simulink model "vehicle_steering"  (R2022a)
settings: Solver=VariableStepAuto  StartTime=0.0  StopTime=10  RelTol=1e-3
model workspace (MATLAB code in the model file):
  | a = 0.5;
  | b = 1;
  | A = [0, 1; 0, 0];
  | B = [a/b; 1];
  | C = [1, 0];
  | D = 0;
  | 
  | P = [-5, -5];
  | % P = [-50, -50];
  | 
  | kr = 23;
  | % kr = 2300;
  | % kr = 90;
  | K = acker(A, B, P);
  | L = [100; 1000]; % from hit and trial
settings Model: Creator=ba13  LastModifiedBy=ba13
settings DataIOCC: Refine=100

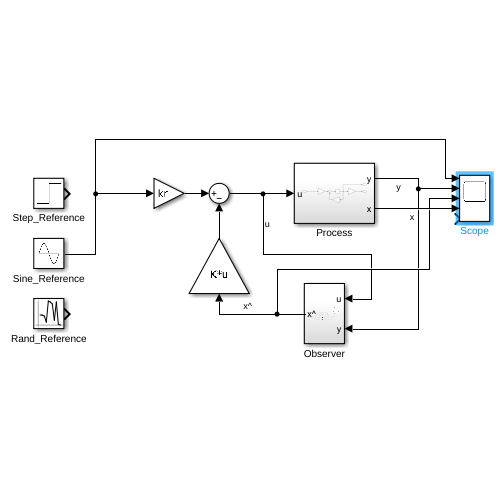
[thumbnail: Simulink's stored preview of the top-level diagram]
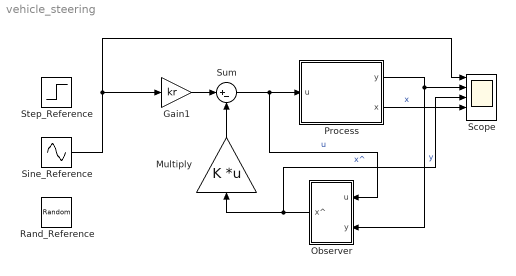
== system vehicle_steering ==
  Gain1 : Gain  Gain=kr
  Multiply : Gain  Gain=K  Multiplication=Matrix(K*u)
  Observer : Subsystem
  Process : Subsystem
  Rand_Reference : RandomNumber  Variance=4  SampleTime=1
  Scope : Scope  NumInputPorts=5
  Sine_Reference : Sin  Amplitude=2  Frequency=2  Phase=1  SampleTime=0
  Step_Reference : Step  After=2  SampleTime=0
  Sum : Sum  Inputs=|+-
  wires:
  Gain1/1 -> Sum/1
  Multiply/1 -> Sum/2
  Sum/1 -> Observer/1(u), Process/1(u)  "u"
  Process/1(y) -> Observer/2(y), Scope/2  "y"
  Observer/1(x^) -> Scope/3, Multiply/1  "x^"
  Process/2(x) -> Scope/4  "x"
  Sine_Reference/1 -> Gain1/1, Scope/1

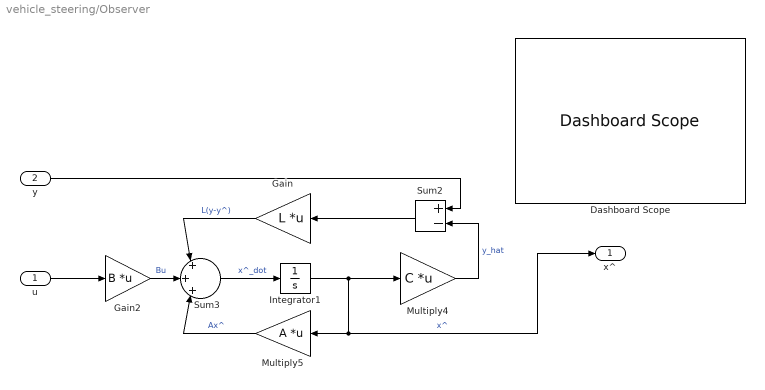
== system vehicle_steering/Observer ==
  u : Inport
  y : Inport  Port=2
  Dashboard Scope : DashboardScope
  Gain : Gain  Gain=L  Multiplication=Matrix(K*u)
  Gain2 : Gain  Gain=B  Multiplication=Matrix(K*u)
  Integrator1 : Integrator
  Multiply4 : Gain  Gain=C  Multiplication=Matrix(K*u)
  Multiply5 : Gain  Gain=A  Multiplication=Matrix(K*u)
  Sum2 : Sum  Inputs=+-
  Sum3 : Sum  Inputs=|+|+|+|
  x^ : Outport
  wires:
  Gain2/1 -> Sum3/2  "Bu"
  Multiply4/1 -> Sum2/2  "y_hat"
  u/1 -> Gain2/1
  Gain/1 -> Sum3/1  "L(y-y^)"
  Sum3/1 -> Integrator1/1  "x^_dot"
  Multiply5/1 -> Sum3/3  "Ax^"
  Sum2/1 -> Gain/1
  Integrator1/1 -> Multiply5/1, x^/1, Multiply4/1  "x^"
  y/1 -> Sum2/1

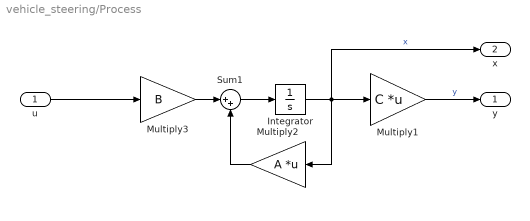
== system vehicle_steering/Process ==
  u : Inport
  Integrator : Integrator
  Multiply1 : Gain  Gain=C  Multiplication=Matrix(K*u)
  Multiply2 : Gain  Gain=A  Multiplication=Matrix(K*u)
  Multiply3 : Gain  Gain=B
  Sum1 : Sum  Inputs=|++
  y : Outport
  x : Outport  Port=2
  wires:
  Multiply2/1 -> Sum1/2
  Sum1/1 -> Integrator/1
  u/1 -> Multiply3/1
  Integrator/1 -> x/1, Multiply2/1, Multiply1/1  "x"
  Multiply3/1 -> Sum1/1
  Multiply1/1 -> y/1  "y"
